simulink model "mpc_mil"  (R2024b)
settings: Solver=ode1  StartTime=0  StopTime=10  FixedStep=0.001  RelTol=1e-3
libraries: Solver_SF x1, simulink x1
settings Model: Creator=user  LastModifiedBy=user
settings OptimizationCC: ZeroExternalMemoryAtStartup=off  ZeroInternalMemoryAtStartup=off
settings RTWCC: TargetLang=C++
settings GRTTargetCC: TargetLangStandard=C++11 (ISO)  CodeInterfacePackaging=C++ class

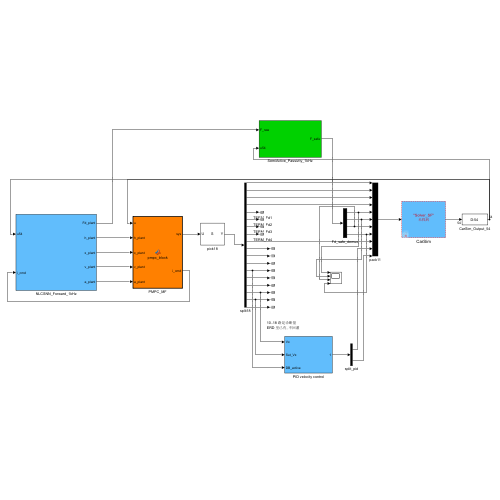
[thumbnail: Simulink's stored preview of the top-level diagram]
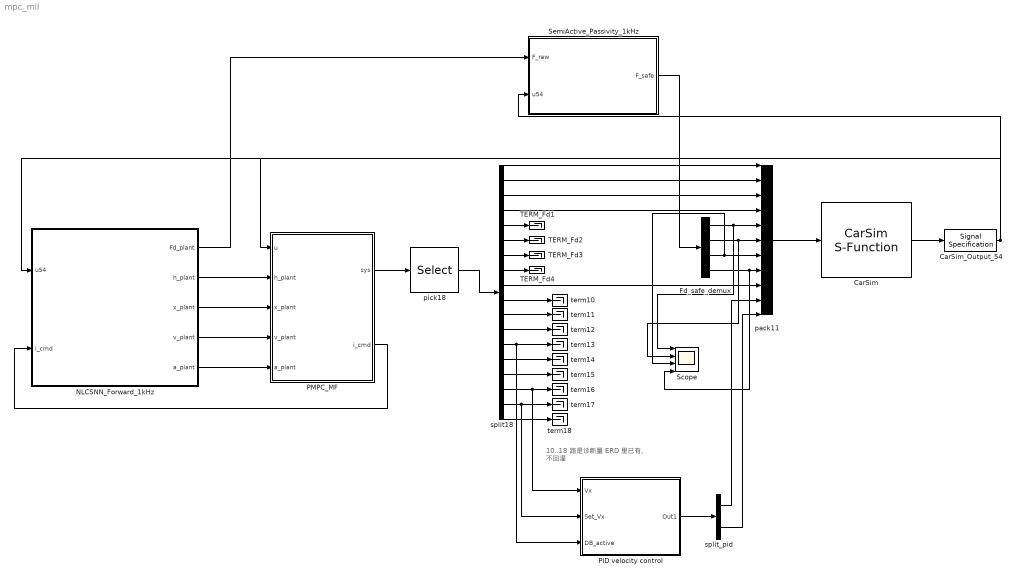
== system mpc_mil ==
  note: 10..18 路是诊断量
      | ERD 里已有, 不回灌
  CarSim : Solver_SF/CarSim S-Function  Priority=1  SIMFILE=simfile.sim
  CarSim_Output_54 : SignalSpecification  Dimensions=54
  Fd_safe_demux : Demux
  NLCSNN_Forward_1kHz : Subsystem
  PID velocity control : Subsystem
  PMPC_MF : MATLAB Function  TreatAsAtomicUnit=on
  Scope : Scope  NumInputPorts=4
  SemiActive_Passivity_1kHz : Subsystem
  TERM_Fd{1..4} (4 alike) : Terminator
  pack11 : Mux  Inputs=11
  pick18 : Selector  InputPortWidth=54  IndexOptions=Index vector (dialog)  Indices=[1 2 3 4 5 6 7 8 9 14 15 16 21 29 30 31 32 38]  OutputSizes=1
  split18 : Demux  Outputs=18
  split_pid : Demux  Outputs=2
  term{10..18} (9 alike) : Terminator
  wires:
  PMPC_MF/1(sys) -> pick18/1
  pick18/1 -> split18/1
  split18/13 -> term13/1, PID velocity control/3(DB_active)
  split18/16 -> term16/1, PID velocity control/1(Vx)
  split18/17 -> term17/1, PID velocity control/2(Set_Vx)
  PID velocity control/1(Out1) -> split_pid/1
  split18/1 -> pack11/1
  split18/2 -> pack11/2
  split18/3 -> pack11/3
  split18/4 -> pack11/4
  split18/9 -> pack11/9
  split18/10 -> term10/1
  split18/11 -> term11/1
  split18/12 -> term12/1
  split18/14 -> term14/1
  split18/15 -> term15/1
  split18/18 -> term18/1
  split_pid/1 -> pack11/10
  split_pid/2 -> pack11/11
  pack11/1 -> CarSim/1
  split18/5 -> TERM_Fd1/1
  split18/6 -> TERM_Fd2/1
  split18/7 -> TERM_Fd3/1
  split18/8 -> TERM_Fd4/1
  PMPC_MF/2(i_cmd) -> NLCSNN_Forward_1kHz/2(i_cmd)
  NLCSNN_Forward_1kHz/2(h_plant) -> PMPC_MF/2(h_plant)
  NLCSNN_Forward_1kHz/3(x_plant) -> PMPC_MF/3(x_plant)
  NLCSNN_Forward_1kHz/4(v_plant) -> PMPC_MF/4(v_plant)
  NLCSNN_Forward_1kHz/5(a_plant) -> PMPC_MF/5(a_plant)
  NLCSNN_Forward_1kHz/1(Fd_plant) -> SemiActive_Passivity_1kHz/1(F_raw)
  SemiActive_Passivity_1kHz/1(F_safe) -> Fd_safe_demux/1
  Fd_safe_demux/1 -> Scope/1, pack11/5
  Fd_safe_demux/2 -> Scope/2, pack11/6
  Fd_safe_demux/3 -> Scope/3, pack11/7
  Fd_safe_demux/4 -> Scope/4, pack11/8
  CarSim/1 -> CarSim_Output_54/1
  CarSim_Output_54/1 -> PMPC_MF/1(u), NLCSNN_Forward_1kHz/1(u54), SemiActive_Passivity_1kHz/2(u54)

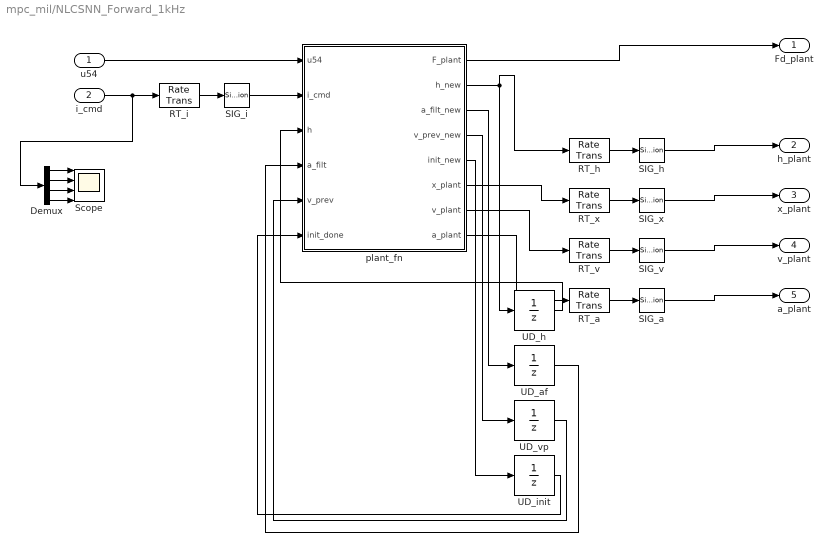
== system mpc_mil/NLCSNN_Forward_1kHz ==
  u54 : Inport
  i_cmd : Inport  Port=2
  Demux : Demux
  RT_a : RateTransition
  RT_h : RateTransition
  RT_i : RateTransition
  RT_v : RateTransition
  RT_x : RateTransition
  SIG_a : SignalSpecification  Dimensions=[4 1]
  SIG_h : SignalSpecification  Dimensions=[8 4]
  SIG_i : SignalSpecification  Dimensions=4
  SIG_v : SignalSpecification  Dimensions=[4 1]
  SIG_x : SignalSpecification  Dimensions=[4 1]
  Scope : Scope  NumInputPorts=4
  UD_af : UnitDelay  InitialCondition=zeros(4,1)  SampleTime=0.001  HasFrameUpgradeWarning=on
  UD_h : UnitDelay  InitialCondition=zeros(8,4)  SampleTime=0.001  HasFrameUpgradeWarning=on
  UD_init : UnitDelay  SampleTime=0.001  HasFrameUpgradeWarning=on
  UD_vp : UnitDelay  InitialCondition=zeros(4,1)  SampleTime=0.001  HasFrameUpgradeWarning=on
  plant_fn : MATLAB Function  TreatAsAtomicUnit=on
  Fd_plant : Outport
  h_plant : Outport  Port=2
  x_plant : Outport  Port=3
  v_plant : Outport  Port=4
  a_plant : Outport  Port=5
  wires:
  u54/1 -> plant_fn/1(u54)
  i_cmd/1 -> Demux/1, RT_i/1
  RT_i/1 -> SIG_i/1
  SIG_i/1 -> plant_fn/2(i_cmd)
  UD_h/1 -> plant_fn/3(h)
  UD_af/1 -> plant_fn/4(a_filt)
  UD_vp/1 -> plant_fn/5(v_prev)
  UD_init/1 -> plant_fn/6(init_done)
  plant_fn/2(h_new) -> RT_h/1, UD_h/1
  plant_fn/3(a_filt_new) -> UD_af/1
  plant_fn/4(v_prev_new) -> UD_vp/1
  plant_fn/5(init_new) -> UD_init/1
  plant_fn/1(F_plant) -> Fd_plant/1
  RT_h/1 -> SIG_h/1
  SIG_h/1 -> h_plant/1
  plant_fn/6(x_plant) -> RT_x/1
  RT_x/1 -> SIG_x/1
  SIG_x/1 -> x_plant/1
  plant_fn/7(v_plant) -> RT_v/1
  RT_v/1 -> SIG_v/1
  SIG_v/1 -> v_plant/1
  plant_fn/8(a_plant) -> RT_a/1
  RT_a/1 -> SIG_a/1
  SIG_a/1 -> a_plant/1
  Demux/1 -> Scope/1
  Demux/2 -> Scope/2
  Demux/3 -> Scope/3
  Demux/4 -> Scope/4

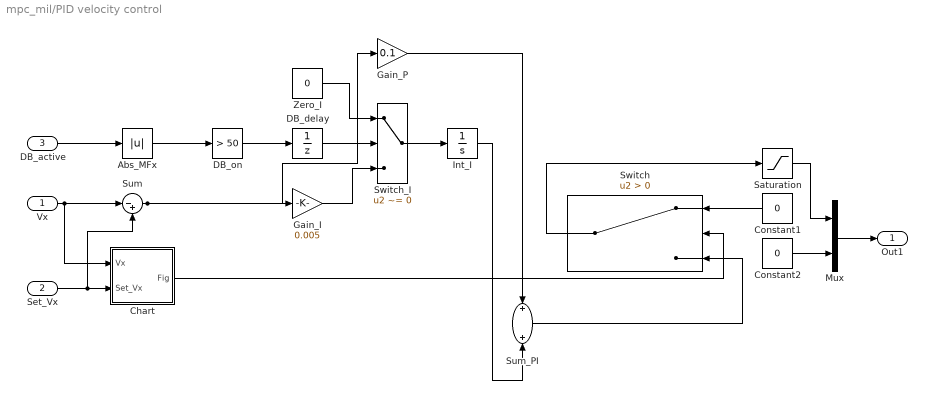
== system mpc_mil/PID velocity control ==
  Vx : Inport
  Set_Vx : Inport  Port=2
  DB_active : Inport  Port=3
  Abs_MFx : Abs  SaturateOnIntegerOverflow=off
  Chart : Stateflow chart  TreatAsAtomicUnit=on
  Constant1 : Constant  Value=0
  Constant2 : Constant  Value=0
  DB_delay : UnitDelay  SampleTime=-1  HasFrameUpgradeWarning=on
  DB_on : simulink/Logic and Bit Operations/Compare To Constant  relop=>  const=50  OutDataTypeStr=uint8
  Gain_I : Gain  Description=2026-09-26: integrand is the signed error e_v = v_tar - v_x (paper IV-D). Before: |e_v| via an Abs block, so the integral kept growing during overspeed (windup).  Gain=0.005
  Gain_P : Gain  Gain=0.1
  Int_I : Integrator
  Mux : Mux  Inputs=2
  Saturation : Saturate  UpperLimit=1  LowerLimit=0
  Sum : Sum  Description=e_v = Set_Vx - Vx (paper IV-D); signs set by port, checked 2026-09-26.  Inputs=|-+
  Sum_PI : Sum
  Switch : Switch  Criteria=u2 > Threshold  SaturateOnIntegerOverflow=off  InputSameDT=off
  Switch_I : Switch  Criteria=u2 ~= 0  SaturateOnIntegerOverflow=off  InputSameDT=off
  Zero_I : Constant  Value=0
  Out1 : Outport
  wires:
  Mux/1 -> Out1/1
  Constant2/1 -> Mux/2
  Switch/1 -> Saturation/1
  Sum_PI/1 -> Switch/3
  Int_I/1 -> Sum_PI/2
  Switch_I/1 -> Int_I/1
  Gain_P/1 -> Sum_PI/1
  Constant1/1 -> Switch/1
  Gain_I/1 -> Switch_I/3
  Zero_I/1 -> Switch_I/1
  Saturation/1 -> Mux/1
  Abs_MFx/1 -> DB_on/1
  DB_on/1 -> DB_delay/1
  Vx/1 -> Sum/1, Chart/1(Vx)
  DB_delay/1 -> Switch_I/2
  DB_active/1 -> Abs_MFx/1
  Set_Vx/1 -> Chart/2(Set_Vx), Sum/2
  Chart/1(Fig) -> Switch/2
  Sum/1 -> Gain_P/1, Gain_I/1

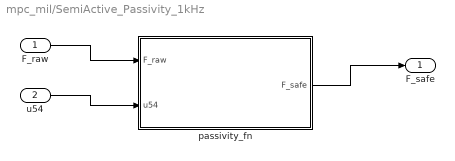
== system mpc_mil/SemiActive_Passivity_1kHz ==
  F_raw : Inport
  u54 : Inport  Port=2
  passivity_fn : MATLAB Function  TreatAsAtomicUnit=on
  F_safe : Outport
  wires:
  ? -> ?
  F_raw/1 -> passivity_fn/1(F_raw)
  u54/1 -> passivity_fn/2(u54)
  passivity_fn/1(F_safe) -> F_safe/1

== matlab function mpc_mil/NLCSNN_Forward_1kHz/plant_fn ==
  settings: updateMethod=DISCRETE  sampleTime=0.001
  data: u54 input; F_plant output; i_cmd input; h input; a_filt input; v_prev input; init_done input; h_new output; a_filt_new output; v_prev_new output; init_new output; x_plant output; v_plant output; a_plant output; NLCSNN parameter
function [F_plant,h_new,a_filt_new,v_prev_new,init_new,x_plant,v_plant,a_plant] = ...
    plant_fn(u54,i_cmd,h,a_filt,v_prev,init_done,NLCSNN)
%#codegen
u54 = reshape(u54,54,1);
i_cmd = reshape(i_cmd,4,1);
h = reshape(h,8,4);
a_filt = reshape(a_filt,4,1);
v_prev = reshape(v_prev,4,1);
cmpRD = u54(1:4);
cmpD = u54(51:54);
[F_plant,h_new,a_filt_new,v_prev_new,init_new,x_plant,v_plant,a_plant] = ...
    func_NLCSNNPlant4(NLCSNN.net,cmpD,cmpRD,i_cmd,h,a_filt,v_prev,init_done,NLCSNN);
end

== matlab function mpc_mil/PMPC_MF ==
  settings: updateMethod=DISCRETE  sampleTime=0.01
  data: u input size=54; h_plant input size=[8 4]; x_plant input size=[4 1]; v_plant input size=[4 1]; a_plant input size=[4 1]; sys output size=54; MPC_P parameter; i_cmd output size=4
function [sys, i_cmd] = mpc_block(u, h_plant, x_plant, v_plant, a_plant, MPC_P) %#codegen
%MPC_BLOCK  Fixed six-state MPC entry point for mpc_mil.

if MPC_P.Pm.MPCParameters.ControllerVariant ~= 1
    error('mpc_block:WrongVariant', 'mpc_block requires ControllerVariant=1.');
end
if numel(u) ~= 54
    error('mpc_block:InvalidInputSize', 'Expected 54 CarSim export channels, received %d.', numel(u));
end

persistent St
if isempty(St)
    St = MPC_P.S0;
end
[sys, St, i_cmd] = pmpc_step(u(:), MPC_P.Pm, St, ...
    h_plant, x_plant, v_plant, a_plant);
end

== stateflow chart mpc_mil/PID velocity control/Chart ==
  (default) -> (junction 4)
  (junction 4) -> (junction 7) [order 2] : [Vx>=Set_Vx]
  (junction 4) -> (junction 6) [order 1] : [Vx<Set_Vx]{Fig=-1;}
  (junction 7) -> (junction 11)
  (junction 11) -> (junction 13) [order 1] : [Vx>Set_Vx]{Fig=1;}
  (junction 11) -> (junction 15) [order 2] : [Vx==Set_Vx]{Fig=0;}
  (junction 13) -> (junction 17)
  (junction 15) -> (junction 6)
  (junction 17) -> (junction 15)
  data: Vx input double; Set_Vx input double; Fig output

== matlab function mpc_mil/SemiActive_Passivity_1kHz/passivity_fn ==
  settings: updateMethod=DISCRETE  sampleTime=0.001
  data: F_raw input; F_safe output; u54 input; NLCSNN parameter
function F_safe = passivity_fn(F_raw,u54,NLCSNN)
%#codegen
F_raw = reshape(F_raw,4,1);
u54 = reshape(u54,54,1);
cmpRD = u54(1:4);
F_safe = func_SemiActivePassivity(F_raw,cmpRD,NLCSNN.passivity);
end
